simulink model "Sim_Modell_RFJ"  (R2020b)
settings: Solver=VariableStepAuto  StartTime=0.0  StopTime=10.0  RelTol=1e-3
undefined symbols (not defined in the file or in its folder): ACD120_80_Rotor, ACD120_80_Stator, Ausleger, Auslegerplatte, DistanzhuelseGP, Federbolzen, Grundplatte, Heidenhain_ERN_1080, Lagerdeckel_oben, Lagerdeckel_unten, par_imp, parSys, Seitenplatte, Visualisierung, Welle, X, Y, Z
libraries: sm_lib x37, fl_lib x7, nesl_utility x7, cstblocks x2, simulink x1
(part 1 of 3)
settings Model: Creator=ukn  LastModifiedBy=ukn

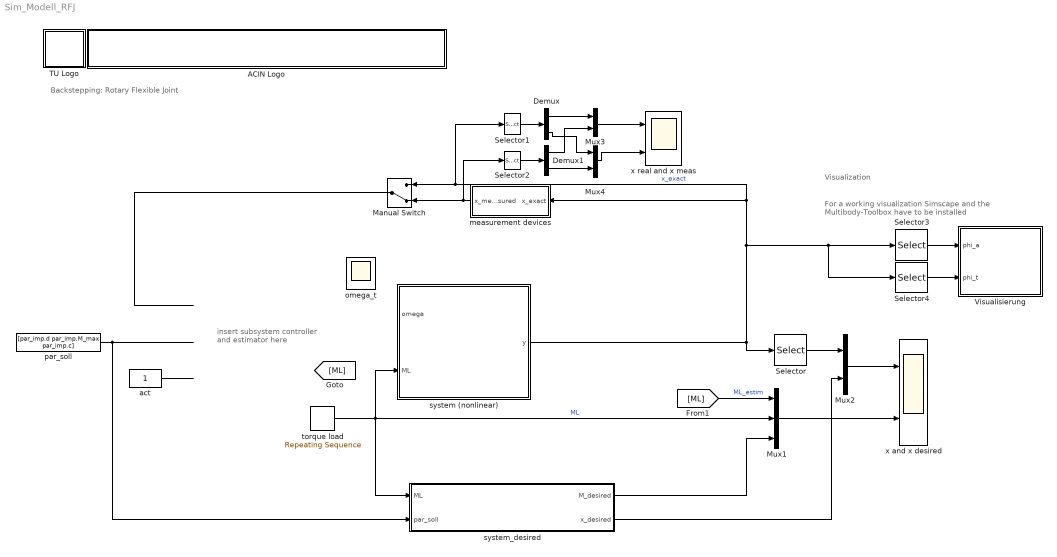
== system Sim_Modell_RFJ ==
  note: For a working visualization Simscape and
      | the Multibody-Toolbox have to be installed
  note: Backstepping: Rotary Flexible Joint
  note: Visualization
  note: insert subsystem
      | controller and
      | estimator here
  ACIN Logo : Subsystem
      mask init:
      | s = get_param(gcb,'UserData');
      mask Display:
      | image(s.logo,[0 0 439 45]);
      | %axis image
  Demux : Demux  Outputs=2
  Demux1 : Demux  Outputs=2
  Manual Switch : ManualSwitch  CurrentSetting=0
  Mux1 : Mux  Inputs=3
  Mux2 : Mux  Inputs=2
  Mux3 : Mux  Inputs=2
  Mux4 : Mux  Inputs=2
  Selector : Selector  InputPortWidth=3  IndexOptions=Index vector (dialog)  Indices=[1 2]  OutputSizes=1
  Selector1 : Selector  InputPortWidth=3  IndexOptions=Index vector (dialog)  Indices=[1 2]  OutputSizes=1
  Selector2 : Selector  InputPortWidth=3  IndexOptions=Index vector (dialog)  Indices=[1 2]  OutputSizes=1
  Selector3 : Selector  InputPortWidth=3  IndexOptions=Index vector (dialog)  Indices=[1]  OutputSizes=1
  Selector4 : Selector  InputPortWidth=3  IndexOptions=Index vector (dialog)  Indices=[3]  OutputSizes=1
  TU Logo : Subsystem
      mask init:
      | s = get_param(gcb,'UserData');
      mask Display: image(s.logo,[0 0 45 45]);
  Visualisierung : Subsystem
  act : Constant
  measurement devices : Subsystem
  omega_t : Scope
  par_soll : Constant  Value=[par_imp.d par_imp.M_max par_imp.c]
  system (nonlinear) : Subsystem
      mask Display: image('$imagefile'); % Use "Edit Image" on toolstrip to change.
  system_desired : Subsystem
      mask init:
      | resources = get_param(gcb,'UserData');
      mask Display:
      | image(resources.logo);
      | port_label('output', 1, 'M_desired');
      | port_label('output', 2, 'x_desired');
      | port_label('input', 1, 'ML');
      | port_label('input', 2, 'par_soll');
  torque load : simulink/Sources/Repeating Sequence  rep_seq_t=[0 0.5 1 1.5 1.50001 5]  rep_seq_y=[0 0 1 1 0 0]*0.1
  x and x desired : Scope  NumInputPorts=2
  x real and x meas : Scope  NumInputPorts=2
  wires:
  system (nonlinear)/1(y) -> Selector/1, Selector4/1, Selector3/1, measurement devices/1(x_exact), Manual Switch/1, Selector1/1  "x_exact"
  Manual Switch/1 -> ?
  Demux1/1 -> Mux3/2
  act/1 -> ?
  measurement devices/1(x_measured) -> Manual Switch/2, Selector2/1
  Mux3/1 -> x real and x meas/1
  Demux/2 -> Mux4/1
  par_soll/1 -> system_desired/2(par_soll)
  torque load/1 -> system (nonlinear)/2(ML), Mux1/2, system_desired/1(ML)  "ML"
  system_desired/1(M_desired) -> Mux1/3
  Mux2/1 -> x and x desired/1
  Selector1/1 -> Demux/1
  system_desired/2(x_desired) -> Mux2/2
  Mux4/1 -> x real and x meas/2
  Mux1/1 -> x and x desired/2
  Demux/1 -> Mux3/1
  ? -> omega_t/1, system (nonlinear)/1(omega)  "u"
  [ML] -> Mux1/1  "ML_estim"
  Selector/1 -> Mux2/1
  Selector2/1 -> Demux1/1
  Demux1/2 -> Mux4/2
  ? -> [ML]
  Selector3/1 -> Visualisierung/1(phi_a)
  Selector4/1 -> Visualisierung/2(phi_t)

== system Sim_Modell_RFJ/ACIN Logo ==

== system Sim_Modell_RFJ/TU Logo ==
